simulink model "modi1_8"  (R2022b)
settings: Solver=VariableStepAuto  StartTime=0.0  StopTime=100.0  RelTol=1e-3
values from neighbouring files (symbols this model uses):
  a0 = 0.00447127    [modi1.m]
  a1 = 0.108205    [modi1.m]
  a2 = 0.683702    [modi1.m]
  alfa1 = 1.2    [modi1.m]
  alfa2 = 0.56    [modi1.m]
  alfa3 = -1.45    [modi1.m]
  alfa4 = 1.15    [modi1.m]
  b0 = 0.00201207    [modi1.m]
  T = 2.5    [modi1.m]
settings Model: Creator=zalew  LastModifiedBy=zalew

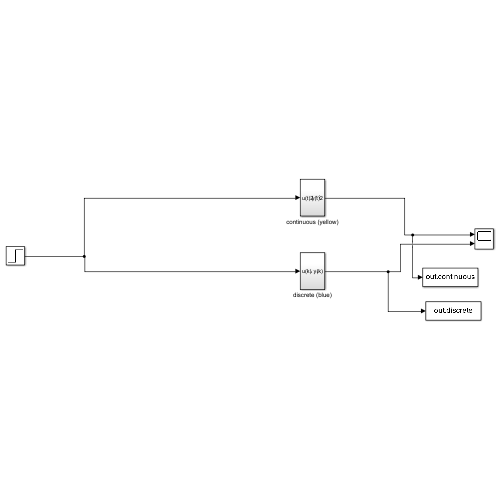
[thumbnail: Simulink's stored preview of the top-level diagram]
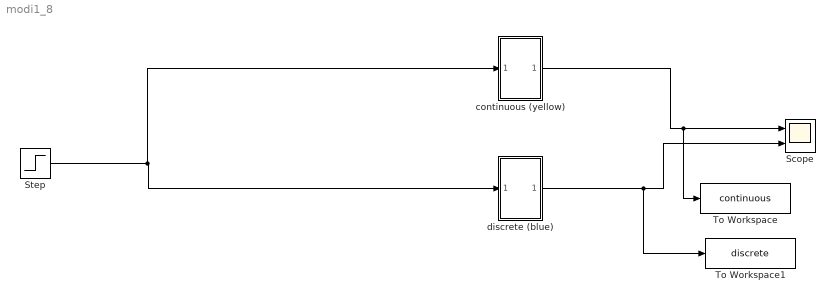
== system modi1_8 ==
  Scope : Scope  NumInputPorts=2
  Step : Step  Time=10  After=0.4  SampleTime=0
  To Workspace : ToWorkspace  VariableName=continuous  SaveFormat=Timeseries  SampleTime=-1
  To Workspace1 : ToWorkspace  VariableName=discrete  SaveFormat=Timeseries  SampleTime=-1
  continuous (yellow) : Subsystem
  discrete (blue) : Subsystem
  wires:
  Step/1 -> continuous (yellow)/1(u(t)2), discrete (blue)/1(u(k))
  discrete (blue)/1(y(k)) -> To Workspace1/1, Scope/2
  continuous (yellow)/1(y(t)2) -> To Workspace/1, Scope/1

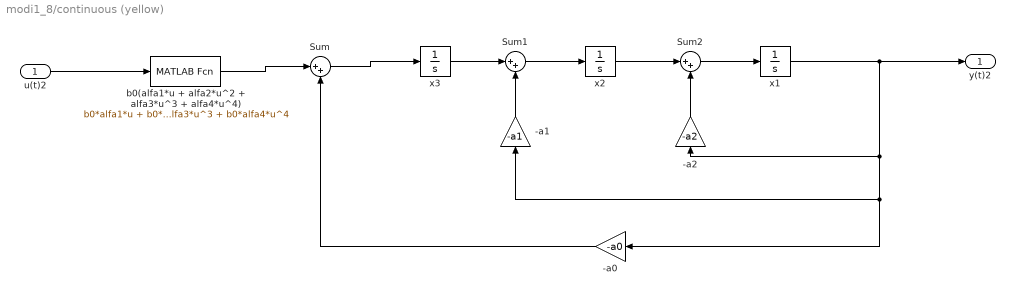
== system modi1_8/continuous (yellow) ==
  u(t)2 : Inport
  -a0 : Gain  Gain=-a0
  -a1 : Gain  Gain=-a1
  -a2 : Gain  Gain=-a2
  Sum : Sum  Inputs=|++
  Sum1 : Sum  Inputs=|++
  Sum2 : Sum  Inputs=|++
  b0(alfa1*u + alfa2*u^2 + alfa3*u^3 + alfa4*u^4) : MATLABFcn  MATLABFcn=b0*alfa1*u + b0*alfa2*u^2 + b0*alfa3*u^3 + b0*alfa4*u^4
  x1 : Integrator
  x2 : Integrator
  x3 : Integrator
  y(t)2 : Outport
  wires:
  -a1/1 -> Sum1/2
  b0(alfa1*u + alfa2*u^2 + alfa3*u^3 + alfa4*u^4)/1 -> Sum/1
  Sum1/1 -> x2/1
  x1/1 -> y(t)2/1, -a2/1, -a1/1, -a0/1
  -a0/1 -> Sum/2
  Sum/1 -> x3/1
  u(t)2/1 -> b0(alfa1*u + alfa2*u^2 + alfa3*u^3 + alfa4*u^4)/1
  -a2/1 -> Sum2/2
  Sum2/1 -> x1/1
  x3/1 -> Sum1/1
  x2/1 -> Sum2/1

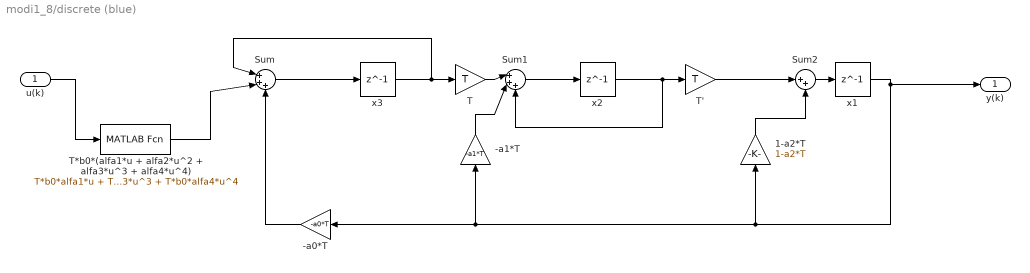
== system modi1_8/discrete (blue) ==
  u(k) : Inport
  -a0*T : Gain  Gain=-a0*T
  -a1*T : Gain  Gain=-a1*T
  1-a2*T : Gain  Gain=1-a2*T
  Sum : Sum  Inputs=|+++
  Sum1 : Sum  Inputs=|+++
  Sum2 : Sum  Inputs=|++
  T : Gain  Gain=T
  T' : Gain  Gain=T
  T*b0*(alfa1*u + alfa2*u^2 + alfa3*u^3 + alfa4*u^4) : MATLABFcn  MATLABFcn=T*b0*alfa1*u + T*b0*alfa2*u^2 + T*b0*alfa3*u^3 + T*b0*alfa4*u^4
  x1 : Delay  DelayLength=1  InitialCondition=0  SampleTime=T
  x2 : Delay  DelayLength=1  InitialCondition=0  SampleTime=T
  x3 : Delay  DelayLength=1  InitialCondition=0  SampleTime=T
  y(k) : Outport
  wires:
  T/1 -> Sum1/1
  x1/1 -> y(k)/1, -a0*T/1, -a1*T/1, 1-a2*T/1
  u(k)/1 -> T*b0*(alfa1*u + alfa2*u^2 + alfa3*u^3 + alfa4*u^4)/1
  1-a2*T/1 -> Sum2/2
  x2/1 -> T'/1, Sum1/3
  Sum1/1 -> x2/1
  T'/1 -> Sum2/1
  Sum/1 -> x3/1
  -a1*T/1 -> Sum1/2
  x3/1 -> Sum/1, T/1
  T*b0*(alfa1*u + alfa2*u^2 + alfa3*u^3 + alfa4*u^4)/1 -> Sum/2
  Sum2/1 -> x1/1
  -a0*T/1 -> Sum/3
